simulink model "massa_molla"  (R2013b)
settings: Solver=ode113  StartTime=0.0  StopTime=10.0  RelTol=1e-5
settings Model: Creator=training-it  LastModifiedBy=training-it
settings SolverCC: ZeroCrossAlgorithm=Adaptive

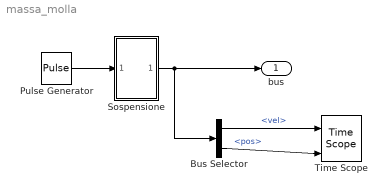
== system massa_molla ==
  Bus Selector : BusSelector  OutputSignals=vel,pos
  Pulse Generator : DiscretePulseGenerator  PulseType=Time based  Period=10  PulseWidth=5
  Sospensione : Subsystem
  Time Scope : TimeScope  NumInputPorts=2  DefaultConfigurationName=spbscopes.TimeScopeBlockCfg
      settings: CopyFcn=scopeextensions.ScopeBlock.onCoreBlockCopy(gcbh);  DeleteFcn=scopeextensions.ScopeBlock.callback(gcbh, 'onBlockDelete');  PreSaveFcn=scopeextensions.ScopeBlock.callback(gcbh, 'onModelSave');  NameChangeFcn=scopeextensions.ScopeBlock.callback(gcbh, 'onBlockRename');  DestroyFcn=scopeextensions.ScopeBlock.onBlockDestroy(gcbh)  CloseFcn=scopeextensions.ScopeBlock.callback(gcbh, 'onBlockClose');  PreDeleteFcn=scopeextensions.ScopeBlock.callback(gcbh, 'onBlockPreDelete');
  bus : Outport
  wires:
  Pulse Generator/1 -> Sospensione/1(In1)
  Sospensione/1(Out1) -> Bus Selector/1, bus/1
  Bus Selector/1 -> Time Scope/1  "<vel>"
  Bus Selector/2 -> Time Scope/2  "<pos>"

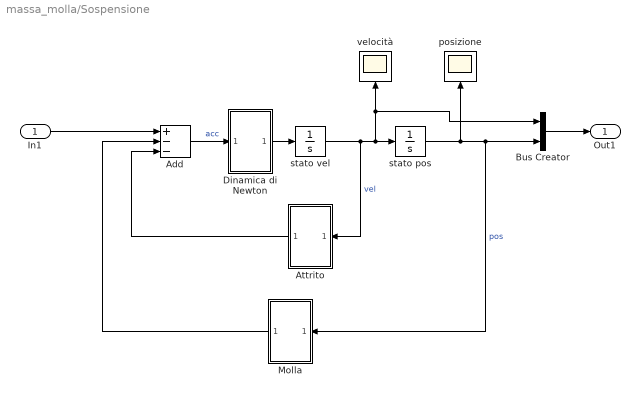
== system massa_molla/Sospensione ==
  In1 : Inport
  Add : Sum  Inputs=+--
  Attrito : Subsystem  mask{c=2}
      mask prompts: c "coeff attrito"
  Bus Creator : BusCreator  Inputs=2
  Dinamica di Newton : Subsystem  mask{m=2}
      mask prompts: m "mass"
  Molla : Subsystem  mask{k=100}
      mask prompts: k "coeff elastico"
  posizione : Scope
  stato pos : Integrator  InitialCondition=x0  mask{x0=0}
      mask prompts: x0 "posizione iniziale"
  stato vel : Integrator  mask{v0=0}
      mask prompts: v0 "velocità iniziale"
  velocità : Scope
  Out1 : Outport
  wires:
  stato pos/1 -> Bus Creator/2, Molla/1(In1), posizione/1  "pos"
  Attrito/1(Out1) -> Add/3
  Molla/1(Out1) -> Add/2
  In1/1 -> Add/1
  Add/1 -> Dinamica di Newton/1(In1)  "acc"
  stato vel/1 -> Attrito/1(In1), velocità/1, Bus Creator/1, stato pos/1  "vel"
  Dinamica di Newton/1(Out1) -> stato vel/1
  Bus Creator/1 -> Out1/1

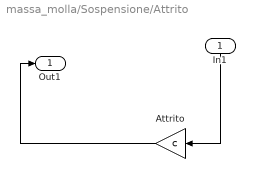
== system massa_molla/Sospensione/Attrito ==
  In1 : Inport
  Attrito : Gain  Gain=c
  Out1 : Outport
  wires:
  Attrito/1 -> Out1/1
  In1/1 -> Attrito/1

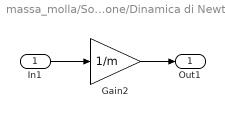
== system massa_molla/Sospensione/Dinamica di Newton ==
  In1 : Inport
  Gain2 : Gain  Gain=1/m
  Out1 : Outport
  wires:
  Gain2/1 -> Out1/1
  In1/1 -> Gain2/1

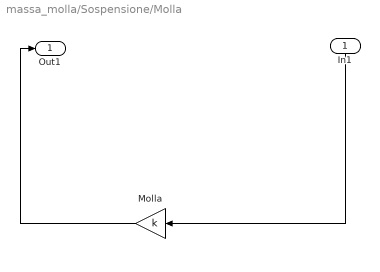
== system massa_molla/Sospensione/Molla ==
  In1 : Inport
  Molla : Gain  Gain=k
  Out1 : Outport
  wires:
  Molla/1 -> Out1/1
  In1/1 -> Molla/1
